simulink model "MealyMoore"  (R2022a)
settings: Solver=FixedStepAuto  StartTime=0.0  StopTime=15.0  RelTol=1e-3
settings Model: Creator=mluser  LastModifiedBy=casti
settings SolverCC: PositivePriorityOrder=on
settings OptimizationCC: EnhancedBackFolding=on  PassReuseOutputArgsAs=Individual arguments  ZeroExternalMemoryAtStartup=off  ZeroInternalMemoryAtStartup=off  MaxStackSize=64  OptimizeBlockOrder=speed  DifferentSizesBufferReuse=on  OptimizationCustomize=off  EfficientTunableParamExpr=on
settings DebuggingCC: ParameterTunabilityLossMsg=error  UnconnectedInputMsg=warning  UnconnectedOutputMsg=warning  UnconnectedLineMsg=warning
settings HardwareCC: ProdBitPerPointer=32  ProdBitPerSizeT=32  ProdBitPerPtrDiffT=32  ProdLargestAtomicInteger=Long  ProdLargestAtomicFloat=Double  ProdWordSize=32  ProdLongLongMode=on  ProdHWDeviceType=ARM Compatible->ARM Cortex
settings RTWCC: SystemTargetFile=ert.tlc  HardwareBoard=Raspberry Pi  TLCOptions="-aInlineSetEventsForThisBaseRateFcn=TLC_FALSE -aSuppressMultiTaskScheduler=TLC_FALSE  -aRateBasedStepFcn=0"  GenCodeOnly=on  TemplateMakefile=ert_default_tmf  GenerateReport=on  Toolchain=GNU GCC Embedded Linux  BuildConfiguration=Faster Runs  IncludeHyperlinkInReport=on  LaunchReport=on  GenerateTraceInfo=on  GenerateTraceReportSl=on  GenerateTraceReportSf=on  DLArmComputeVersion=19.05
settings CodeAppCC: ForceParamTrailComments=on  IgnoreCustomStorageClasses=off  OperatorAnnotations=on  SimulinkDataObjDesc=on  SFDataObjDesc=on  InsertBlockDesc=on
settings ERTTargetCC: SupportVariableSizeSignals=on  ExtModeTransport=2  ExtModeStaticAlloc=on  ExtModeMexFile=ext_xcp  ExtModeIntrfLevel=Level2 - Open

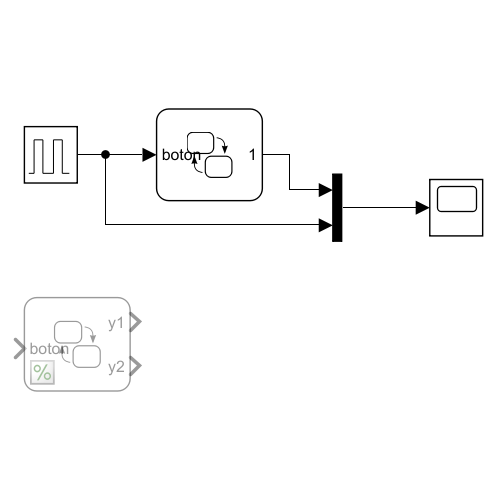
[thumbnail: Simulink's stored preview of the top-level diagram]
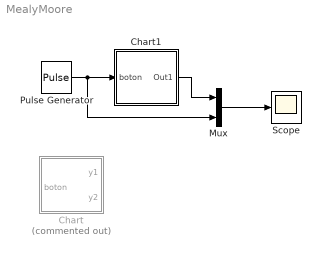
== system MealyMoore ==
  Chart : Stateflow chart  Commented=on  TreatAsAtomicUnit=on
  Chart1 : Stateflow chart  TreatAsAtomicUnit=on
  Mux : Mux  Inputs=2
  Pulse Generator : DiscretePulseGenerator  PulseType=Time based  Period=10  PulseWidth=5  PhaseDelay=1
  Scope : Scope
  wires:
  Pulse Generator/1 -> Mux/2, Chart1/1(boton)
  Mux/1 -> Scope/1
  Chart1/1(Out1) -> Mux/1

== stateflow chart MealyMoore/Chart1 ==
  state Off
    Out1=0
  state On
    Out1=1
  (default) -> Off
  Off -> On : [boton==1]
  data: boton input; Out1 output

== stateflow chart MealyMoore/Chart ==
  state Vehiculos [parallel]
    settings: executionOrder=1
    state Rojo
      y1 = 0
    state Ambar
      y1 = 2
    state Verde
      y1 = 1
    (default) -> Vehiculos.Rojo
    Ambar -> Vehiculos.Rojo : after(10,sec) {send(cambiaARV, Peatonal)}
    Vehiculos.Rojo -> Vehiculos.Verde : after(20,sec){send(cambiaRVV,Peatonal)}
    Vehiculos.Verde -> Ambar [order 1] : [boton == 1]
    Vehiculos.Verde -> Ambar [order 2] : after(30,sec)
  state Peatonal [parallel]
    settings: executionOrder=2
    state Rojo
      y2 = 3
    state Verde
      y2 = 4
    (default) -> Peatonal.Verde
    Peatonal.Verde -> Peatonal.Rojo : cambiaRVV
    Peatonal.Rojo -> Peatonal.Verde : cambiaARV
  data: boton input; y1 output; y2 output
  events: cambiaRVV local FUNCTION_CALL_EVENT; cambiaARV local FUNCTION_CALL_EVENT
